simulink model "LED_Cmd_varZ_testHarness"  (Simulink 8.0)
settings: Solver=FixedStepDiscrete  StartTime=0.0  StopTime=10  RelTol=1e-3
PreLoadFcn:
  | LED_Cmd_varZ_selfinit
InitFcn:
  | sldvharnessinit(6, '');
undefined symbols (not defined in the file): sigbuilder_block
CloseFcn:
  | rtwprivate ssgencode ModelCloseRequest ADL
settings Model: MinMaxOverflowLogging=ForceOff  SldvGeneratedHarnessModel=TestUnitModel=LED_Cmd_varZ|  Creator=fguerin  LastModifiedBy=klindqvi  RecordCoverage=on  CovMetricSettings=dcmoe  CovHTMLOptions=-aTS=1 -bRG=1 -bTC=0 -hTR=0 -nFC=0 -scm=1 -bcm=1 -xEv=0  covSaveCumulativeToWorkspaceVar=off  CovSaveSingleToWorkspaceVar=off  CovCumulativeReport=on  CovReportOnPause=off  CovModelRefEnable=off  CovExternalEMLEnable=on
settings DataIOCC: ExternalInput=SIM_LockDoorRequest  LimitDataPoints=off  SignalLoggingSaveFormat=ModelDataLogs  SaveOutput=off  DSMLogging=off  SaveTime=off  SignalLoggingName=logsOut
settings OptimizationCC: InlineParams=on  InlineInvariantSignals=on  EnhancedBackFolding=on  ZeroExternalMemoryAtStartup=off  ZeroInternalMemoryAtStartup=off  EfficientFloat2IntCast=on  OptimizeModelRefInitCode=on  LifeSpan=1
settings DebuggingCC: SignalInfNanChecking=error  SignalRangeChecking=error  ReadBeforeWriteMsg=EnableAllAsError  WriteAfterWriteMsg=EnableAllAsError  WriteAfterReadMsg=EnableAllAsError  AlgebraicLoopMsg=error  ArtificialAlgebraicLoopMsg=error  SaveWithDisabledLinksMsg=error  SaveWithParameterizedLinksMsg=error  CheckExecutionContextPreStartOutputMsg=on  CheckExecutionContextRuntimeOutputMsg=on  BlockPriorityViolationMsg=error  SolverPrmCheckMsg=error  MultiTaskCondExecSysMsg=warning  MultiTaskRateTransMsg=warning  CheckMatrixSingularityMsg=error  IntegerOverflowMsg=error  ParameterUnderflowMsg=error  ParameterPrecisionLossMsg=error  ParameterTunabilityLossMsg=error  UnderSpecifiedDataTypeMsg=warning  VectorMatrixConversionMsg=error  FcnCallInpInsideContextMsg=EnableAllAsWarning  SFcnCompatibilityMsg=error  BusObjectLabelMismatch=error  RootOutportRequireBusObject=error  AssertControl=DisableAll  ModelReferenceIOMsg=error  ModelReferenceIOMismatchMessage=error  ModelReferenceCSMismatchMessage=warning  UnknownTsInhSupMsg=error  ModelReferenceDataLoggingMessage=error  StrictBusMsg=ErrorOnBusTreatedAsVector
settings HardwareCC: ProdLargestAtomicInteger=Long  ProdLargestAtomicFloat=Double  ProdIntDivRoundTo=Zero  ProdEndianess=BigEndian  ProdHWDeviceType=Freescale->MPC5500
settings ModelReferenceCC: ModelReferenceNumInstancesAllowed=Single
settings SFSimCC: SimParseCustomCode=off
settings RTWCC: SystemTargetFile=ert.tlc  TemplateMakefile=ert_default_tmf  Description=Embedded Coder  GenerateReport=on  RTWVerbose=off  ProcessScript=ert_make_rtw_hook  IncludeHyperlinkInReport=on  LaunchReport=on  PortableWordSizes=on  GenerateTraceInfo=on  GenerateTraceReport=on  GenerateTraceReportSl=on  GenerateTraceReportSf=on  GenerateTraceReportEml=on  GenerateCodeMetricsReport=on
settings MATStruct: className=coder.coverage.Bullseye  argsAllComponents=[]  excludedModels=[]  includeReferencedModels=off  includeTopModel=on  enabled=on
settings CodeAppCC: ForceParamTrailComments=on  IgnoreCustomStorageClasses=off  IgnoreTestpoints=on  MangleLength=4  InlinedPrmAccess=Macros  ReqsInCode=on
settings ERTTargetCC: CodeReplacementLibrary=ANSI_C  MultiwordLength=2048  GenerateSampleERTMain=on  SupportAbsoluteTime=off  SupportNonFinite=off  SupportComplex=off  InlinedParameterPlacement=NonHierarchical  ERTCustomFileTemplate=example_file_process.tlc  ConvertIfToSwitch=off  SuppressUnreachableDefaultCases=off
settings ConfigComp: Description=Design Verifier Custom Configuration Component  DVMaxProcessTime=600  DVDisplayUnsatisfiableObjectives=on  DVAutomaticStubbing=off  DVOutputDir=C:\Work\Data\Pilots\P_PSA_ECoder_BenchMark_LaGarenne\source9b\deliverable\trunk\demos\VnV_example\Projects\ADL_Project/Simulink_Test_Generation/ADL_Sim  DVModelCoverageObjectives=MCDC  DVTestSuiteOptimization=CombinedObjectives  DVDataFileName=./Tests/$ModelName$_sldvdata  DVSaveHarnessModel=on  DVHarnessModelFileName=./Tests/$ModelName$_testHarness  DVModelReferenceHarness=on  DVSaveReport=on  DVReportFileName=ADL_Sim_SLDV.html

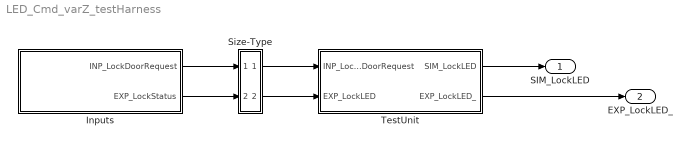
== system LED_Cmd_varZ_testHarness ==
  Inputs : Subsystem  Tag=STV Subsys  RequirementInfo={'other' '..\..\..\..\requirements\doorlockingsystem_swr.doc' '@Simulink_requirement_item_4' 'true' 'REQ202 – The lock mechanism should indicate the state. A locked state should be indicated by a flashing light and an unlocked state by no light.' '' } %GIDa_c42ad1a2_ffa0_475d_b2c2_483f9527a2e0  LoadFcn=sigbuilder_block('load',[508.5 257.25 637.5 399.75 ]);  StartFcn=sigbuilder_block('start');  StopFcn=sigbuilder_block('stop');  ClipboardFcn=sigbuilder_block('clipboard');  mask(Sigbuilder block){}
      mask init:
      | if ~strcmp(get_param(bdroot(gcb),'SimulationStatus'),'stopped'),tuvar = sigbuilder_block('maskInit'); end
      settings: CopyFcn=sigbuilder_block('copy');  DeleteFcn=sigbuilder_block('delete');  ModelCloseFcn=sigbuilder_block('modelClose');  PreSaveFcn=sigbuilder_block('preSave');  PauseFcn=sigbuilder_block('pause')  ContinueFcn=sigbuilder_block('continue')  NameChangeFcn=sigbuilder_block('namechange');  OpenFcn=sigbuilder_block('open',[508.5 257.25 637.5 399.75 ]);  CloseFcn=sigbuilder_block('close');
      mask Display: plot(0, 0, 100, 100,[2, 2, 32, 32, 2], [68, 8, 8, 68, 68],[32, 2], [38, 38], [32, 19, 2],[53, 60, 44], [32, 17, 17, 2],[16, 16, 31, 31]);txt = getActiveGroup(gcbh);text(2, 100, txt,'verticalAlignment', 'top');
  Size-Type : Subsystem
  TestUnit : Subsystem
  SIM_LockLED : Outport
  EXP_LockLED_ : Outport  Port=2
  wires:
  Size-Type/1(Out1) -> TestUnit/1(INP_LockDoorRequest)
  Size-Type/2(Out2) -> TestUnit/2(EXP_LockLED)
  TestUnit/1(SIM_LockLED) -> SIM_LockLED/1
  TestUnit/2(EXP_LockLED_) -> EXP_LockLED_/1
  Inputs/1(INP_LockDoorRequest) -> Size-Type/1(In1)
  Inputs/2(EXP_LockStatus) -> Size-Type/2(In2)

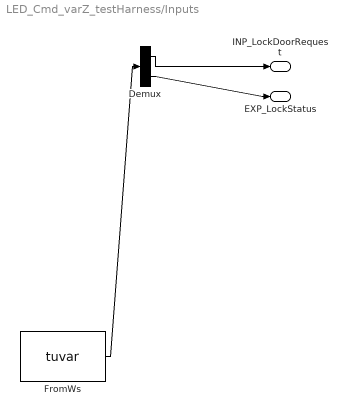
== system LED_Cmd_varZ_testHarness/Inputs ==
  Demux : Demux  Tag=STV Demux  Outputs=2
  FromWs : FromWorkspace  Tag=STV FromWs  VariableName=tuvar  SampleTime=0  SigBuilderData=DataTag0  VnvData=DataTag1
      SigBuilderData=|
      | dataSet(1).timeRange = [0 10]
      | dataSet(1).name = 'Test1'
      | dataSet(2).timeRange = [0 10]
      | dataSet(2).name = 'Test2'
      | dataSet(3).timeRange = [0 10]
      | dataSet(3).name = 'Test3'
      | sbobj.Name = 'Signal Builder'
      | sbobj.Groups(1).Name = 'Test1'
      | sbobj.Groups(1).Signals(1).Name = 'INP_LockDoorRequest'
      | sbobj.Groups(1).Signals(1).XData = [0 10]
      | sbobj.Groups(1).Signals(1).YData = [0 0]
      | sbobj.Groups(1).Signals(2).Name = 'EXP_LockStatus'
      | sbobj.Groups(1).Signals(2).XData = [0 10]
      | sbobj.Groups(1).Signals(2).YData = [0 0]
      | sbobj.Groups(2).Name = 'Test2'
      | sbobj.Groups(2).Signals(1).Name = 'INP_LockDoorRequest'
      | sbobj.Groups(2).Signals(1).XData = [0 1 2 3 4 5 6 7 8 9 10]
      | sbobj.Groups(2).Signals(1).YData = [0 1 1 1 1 1 1 1 1 1 1]
      | sbobj.Groups(2).Signals(2).Name = 'EXP_LockStatus'
      | sbobj.Groups(2).Signals(2).XData = [0 1 2 3 4 5 6 7 8 9 10]
      | sbobj.Groups(2).Signals(2).YData = [0 1 0 1 0 1 0 1 0 1 0]
      | sbobj.Groups(3).Name = 'Test3'
      | sbobj.Groups(3).Signals(1).Name = 'INP_LockDoorRequest'
      | sbobj.Groups(3).Signals(1).XData = [0 1 2 10]
      | sbobj.Groups(3).Signals(1).YData = [0 1 0 0]
      | sbobj.Groups(3).Signals(2).Name = 'EXP_LockStatus'
      | sbobj.Groups(3).Signals(2).XData = [0 1 2 10]
      | sbobj.Groups(3).Signals(2).YData = [0 1 0 0]
  INP_LockDoorRequest : Outport
  EXP_LockStatus : Outport  Tag=STV Outport  Port=2
  wires:
  FromWs/1 -> Demux/1
  Demux/1 -> INP_LockDoorRequest/1
  Demux/2 -> EXP_LockStatus/1

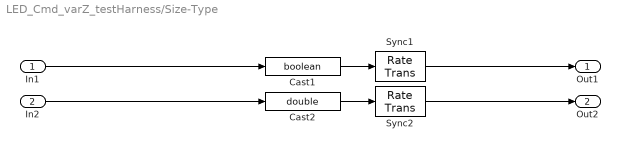
== system LED_Cmd_varZ_testHarness/Size-Type ==
  In1 : Inport
  In2 : Inport  Port=2
  Cast1 : DataTypeConversion  OutDataTypeStr=boolean  SaturateOnIntegerOverflow=on  RndMeth=Zero
  Cast2 : DataTypeConversion  OutDataTypeStr=double  SaturateOnIntegerOverflow=on  RndMeth=Zero
  Sync1 : RateTransition  OutPortSampleTime=1
  Sync2 : RateTransition  OutPortSampleTime=1
  Out1 : Outport
  Out2 : Outport  Port=2
  wires:
  In1/1 -> Cast1/1
  Cast1/1 -> Sync1/1
  Sync1/1 -> Out1/1
  In2/1 -> Cast2/1
  Cast2/1 -> Sync2/1
  Sync2/1 -> Out2/1

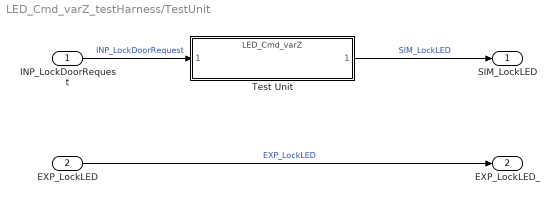
== system LED_Cmd_varZ_testHarness/TestUnit ==
  INP_LockDoorRequest : Inport
  EXP_LockLED : Inport  Port=2
  Test Unit : ModelReference  ModelNameDialog=LED_Cmd_varZ  SimulationMode=Normal  ModelReferenceVersion=1.365  CopyOfModelName=LED_Cmd_varZ  DefaultDataLogging=off
  SIM_LockLED : Outport
  EXP_LockLED_ : Outport  Port=2
  wires:
  EXP_LockLED/1 -> EXP_LockLED_/1  "EXP_LockLED"
  Test Unit/1 -> SIM_LockLED/1  "SIM_LockLED"
  INP_LockDoorRequest/1 -> Test Unit/1  "INP_LockDoorRequest"
